simulink model "bh_test_LINCONT_on_NONLIN_plant"  (R2016a)
settings: Solver=ode23s  StartTime=0.0  StopTime=30  FixedStep=0.001  RelTol=1e-5
undefined symbols (not defined in the file or in its folder): P_one_prop, P_veh, sigbuilder_block
libraries: simulink x6, simulink_extras x5, bh_6dof_LIBRARY x2
settings Model: Creator=bhorton  LastModifiedBy=bhorton
settings DataIOCC: SaveOutput=off  SignalLogging=off  DSMLogging=off  VisualizeSimOutput=off  SaveTime=off
settings DebuggingCC: AllowSymbolicDim=off
settings ModelReferenceCC: PropagateSignalLabelsOutOfModel=off
settings GRTTargetCC: GeneratePreprocessorConditionals=Use local settings

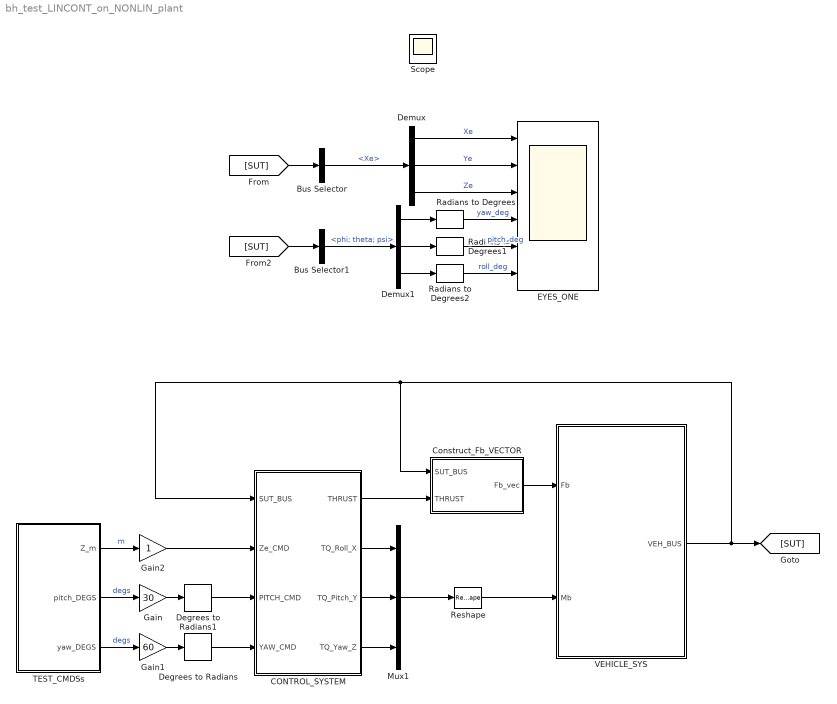
== system bh_test_LINCONT_on_NONLIN_plant ==
  Bus Selector : BusSelector  OutputSignals=Xe
  Bus Selector1 : BusSelector  OutputSignals=phi; theta; psi
  CONTROL_SYSTEM : Subsystem
  Construct_Fb_VECTOR : Subsystem
  Degrees to Radians : simulink_extras/Transformations/Degrees to Radians
  Degrees to Radians1 : simulink_extras/Transformations/Degrees to Radians
  Demux : Demux  Outputs=3
  Demux1 : Demux  Outputs=3
  EYES_ONE : Scope  NumInputPorts=6
  Gain : Gain  Gain=30
  Gain1 : Gain  Gain=60
  Gain2 : Gain
  Mux1 : Mux  Inputs=3
  Radians to Degrees : simulink_extras/Transformations/Radians to Degrees
  Radians to Degrees1 : simulink_extras/Transformations/Radians to Degrees
  Radians to Degrees2 : simulink_extras/Transformations/Radians to Degrees
  Reshape : Reshape  OutputDimensionality=Column vector (2-D)
  TEST_CMDSs : Subsystem  Tag=STV Subsys  LoadFcn=sigbuilder_block('load');  StartFcn=sigbuilder_block('start');  StopFcn=sigbuilder_block('stop');  ClipboardFcn=sigbuilder_block('clipboard');  mask(Sigbuilder block){}
      mask help: Simulink:masks:SigbuilderBlock_MD
      mask init:
      | if ~strcmp(get_param(bdroot(gcbh),'SimulationStatus'),'stopped') tuvar = sigbuilder_block('maskInit'); end
      settings: CopyFcn=sigbuilder_block('copy');  DeleteFcn=sigbuilder_block('delete');  ModelCloseFcn=sigbuilder_block('modelClose');  PreSaveFcn=sigbuilder_block('preSave');  PauseFcn=sigbuilder_block('pause');  ContinueFcn=sigbuilder_block('continue');  NameChangeFcn=sigbuilder_block('namechange');  OpenFcn=sigbuilder_block('open',[140.25 198.75 550.5 399.75 ]);  CloseFcn=sigbuilder_block('close');
      mask Display: plot(0, 0, 100, 100,[2, 2, 32, 32, 2], [68, 8, 8, 68, 68],[32, 2], [38, 38], [32, 19, 2],[53, 60, 44], [32, 17, 17, 2],[16, 16, 31, 31]);txt = getActiveGroup(gcbh);text(2, 100, txt,'verticalAlignment', 'top');
  VEHICLE_SYS : Subsystem
  Scope : Scope
  wires:
  Construct_Fb_VECTOR/1(Fb_vec) -> VEHICLE_SYS/1(Fb)
  Reshape/1 -> VEHICLE_SYS/2(Mb)
  Mux1/1 -> Reshape/1
  TEST_CMDSs/2(pitch_DEGS) -> Gain/1  "degs"
  TEST_CMDSs/1(Z_m) -> Gain2/1  "m"
  TEST_CMDSs/3(yaw_DEGS) -> Gain1/1  "degs"
  Gain/1 -> Degrees to Radians1/1
  Gain1/1 -> Degrees to Radians/1
  Degrees to Radians/1 -> CONTROL_SYSTEM/4(YAW_CMD)
  Degrees to Radians1/1 -> CONTROL_SYSTEM/3(PITCH_CMD)
  CONTROL_SYSTEM/1(THRUST) -> Construct_Fb_VECTOR/2(THRUST)
  CONTROL_SYSTEM/2(TQ_Roll_X) -> Mux1/1
  CONTROL_SYSTEM/3(TQ_Pitch_Y) -> Mux1/2
  CONTROL_SYSTEM/4(TQ_Yaw_Z) -> Mux1/3
  [SUT] -> Bus Selector/1
  Demux/2 -> EYES_ONE/2  "Ye"
  Demux/3 -> EYES_ONE/3  "Ze"
  Demux/1 -> EYES_ONE/1  "Xe"
  Bus Selector/1 -> Demux/1  "<Xe>"
  Bus Selector1/1 -> Demux1/1  "<phi; theta; psi>"
  [SUT] -> Bus Selector1/1
  Demux1/1 -> Radians to Degrees/1
  Radians to Degrees/1 -> EYES_ONE/4  "yaw_deg"
  Radians to Degrees1/1 -> EYES_ONE/5  "pitch_deg"
  Radians to Degrees2/1 -> EYES_ONE/6  "roll_deg"
  Demux1/3 -> Radians to Degrees2/1
  Demux1/2 -> Radians to Degrees1/1
  VEHICLE_SYS/1(VEH_BUS) -> [SUT], CONTROL_SYSTEM/1(SUT_BUS), Construct_Fb_VECTOR/1(SUT_BUS)
  Gain2/1 -> CONTROL_SYSTEM/2(Ze_CMD)

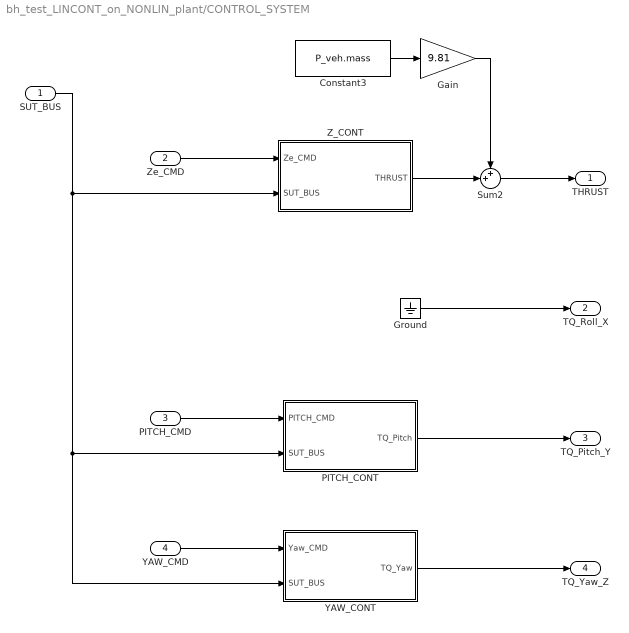
== system bh_test_LINCONT_on_NONLIN_plant/CONTROL_SYSTEM ==
  SUT_BUS : Inport
  Ze_CMD : Inport  Port=2
  PITCH_CMD : Inport  Port=3
  YAW_CMD : Inport  Port=4
  Constant3 : Constant  Value=P_veh.mass
  Gain : Gain  Gain=9.81
  Ground : Ground
  PITCH_CONT : Subsystem
  Sum2 : Sum  Inputs=++|
  YAW_CONT : Subsystem
  Z_CONT : Subsystem
  THRUST : Outport
  TQ_Roll_X : Outport  Port=2
  TQ_Pitch_Y : Outport  Port=3
  TQ_Yaw_Z : Outport  Port=4
  wires:
  SUT_BUS/1 -> PITCH_CONT/2(SUT_BUS), YAW_CONT/2(SUT_BUS), Z_CONT/2(SUT_BUS)
  Ze_CMD/1 -> Z_CONT/1(Ze_CMD)
  PITCH_CMD/1 -> PITCH_CONT/1(PITCH_CMD)
  YAW_CMD/1 -> YAW_CONT/1(Yaw_CMD)
  Z_CONT/1(THRUST) -> Sum2/2
  YAW_CONT/1(TQ_Yaw) -> TQ_Yaw_Z/1
  PITCH_CONT/1(TQ_Pitch) -> TQ_Pitch_Y/1
  Ground/1 -> TQ_Roll_X/1
  Sum2/1 -> THRUST/1
  Gain/1 -> Sum2/1
  Constant3/1 -> Gain/1

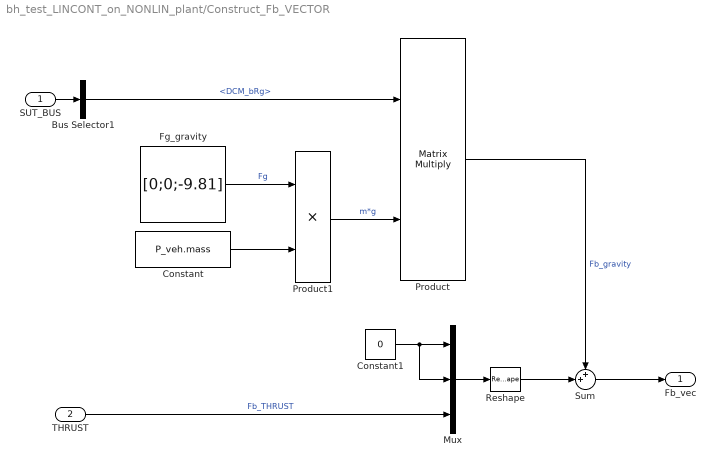
== system bh_test_LINCONT_on_NONLIN_plant/Construct_Fb_VECTOR ==
  SUT_BUS : Inport
  THRUST : Inport  Port=2
  Bus Selector1 : BusSelector  OutputSignals=DCM_bRg
  Constant : Constant  Value=P_veh.mass
  Constant1 : Constant  Value=0
  Fg_gravity : Constant  Value=[0;0;-9.81]  VectorParams1D=off
  Mux : Mux  Inputs=3
  Product : Product  Multiplication=Matrix(*)
  Product1 : Product
  Reshape : Reshape  OutputDimensionality=Column vector (2-D)
  Sum : Sum  Inputs=++|
  Fb_vec : Outport
  wires:
  Mux/1 -> Reshape/1
  Sum/1 -> Fb_vec/1
  SUT_BUS/1 -> Bus Selector1/1
  THRUST/1 -> Mux/3  "Fb_THRUST"
  Constant1/1 -> Mux/2, Mux/1
  Bus Selector1/1 -> Product/1  "<DCM_bRg>"
  Reshape/1 -> Sum/2
  Product/1 -> Sum/1  "Fb_gravity"
  Product1/1 -> Product/2  "m*g"
  Fg_gravity/1 -> Product1/1  "Fg"
  Constant/1 -> Product1/2

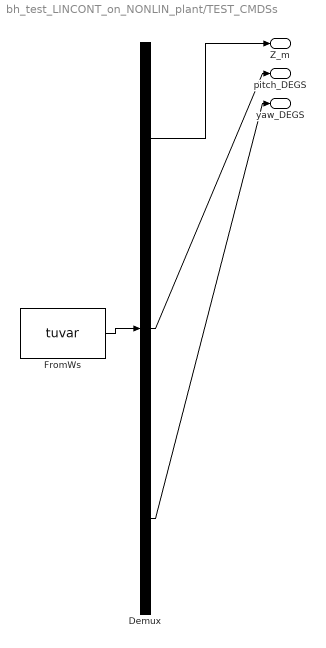
== system bh_test_LINCONT_on_NONLIN_plant/TEST_CMDSs ==
  Demux : Demux  Tag=STV Demux  Outputs=3
  FromWs : FromWorkspace  Tag=STV FromWs  VariableName=tuvar  SampleTime=0
      SigBuilderData=|
      | common.afterFinalStr = 'Extrapolate'
      | common.sampleTime = 0
      | dataSet.timeRange = [0 20]
      | dataSet.name = 'Group 1'
      | sbobj.Groups.Name = 'Group 1'
      | sbobj.Groups.Signals(1).Name = 'Z_m'
      | sbobj.Groups.Signals(1).XData = [0 1 1 6 20]
      | sbobj.Groups.Signals(1).YData = [0 0 1 1 1]
      | sbobj.Groups.Signals(2).Name = 'pitch_DEGS'
      | sbobj.Groups.Signals(2).XData = [0 8 8 10 10 20]
      | sbobj.Groups.Signals(2).YData = [0 0 1 1 0 0]
      | sbobj.Groups.Signals(3).Name = 'yaw_DEGS'
      | sbobj.Groups.Signals(3).XData = [0 13.95 13.95 18 18 20]
      | sbobj.Groups.Signals(3).YData = [0 0 1 1 0 0]
      | sbobj.Groups.TimeRange = [0 20]
  Z_m : Outport  Tag=STV Outport
  pitch_DEGS : Outport  Tag=STV Outport  Port=2
  yaw_DEGS : Outport  Tag=STV Outport  Port=3
  wires:
  Demux/1 -> Z_m/1
  FromWs/1 -> Demux/1
  Demux/2 -> pitch_DEGS/1
  Demux/3 -> yaw_DEGS/1

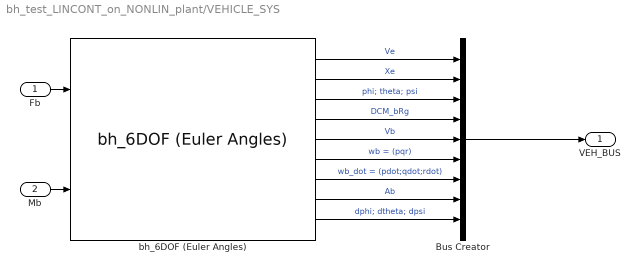
== system bh_test_LINCONT_on_NONLIN_plant/VEHICLE_SYS ==
  Fb : Inport
  Mb : Inport  Port=2
  Bus Creator : BusCreator  Inputs=9
  bh_6DOF (Euler Angles) : bh_6dof_LIBRARY/MODELS/bh_6DOF (Euler Angles)  inertia_0=P_veh.I  mass_0=P_veh.mass  xme_0=P_veh.Xe_init  Vm_0=P_veh.Vb_init  pm_0=P_veh.wb_init  eul_0=P_veh.eul_init
  VEH_BUS : Outport
  wires:
  Fb/1 -> bh_6DOF (Euler Angles)/1
  Mb/1 -> bh_6DOF (Euler Angles)/2
  bh_6DOF (Euler Angles)/3 -> Bus Creator/3  "phi; theta; psi"
  bh_6DOF (Euler Angles)/2 -> Bus Creator/2  "Xe"
  bh_6DOF (Euler Angles)/1 -> Bus Creator/1  "Ve"
  bh_6DOF (Euler Angles)/4 -> Bus Creator/4  "DCM_bRg"
  bh_6DOF (Euler Angles)/8 -> Bus Creator/8  "Ab"
  bh_6DOF (Euler Angles)/7 -> Bus Creator/7  "wb_dot = (pdot;qdot;rdot)"
  Bus Creator/1 -> VEH_BUS/1
  bh_6DOF (Euler Angles)/5 -> Bus Creator/5  "Vb"
  bh_6DOF (Euler Angles)/6 -> Bus Creator/6  "wb = (pqr)"
  bh_6DOF (Euler Angles)/9 -> Bus Creator/9  "dphi; dtheta; dpsi"

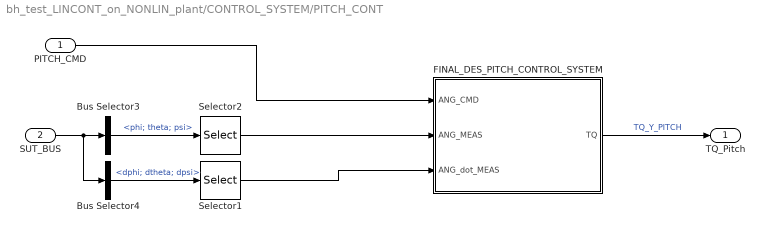
== system bh_test_LINCONT_on_NONLIN_plant/CONTROL_SYSTEM/PITCH_CONT ==
  PITCH_CMD : Inport
  SUT_BUS : Inport  Port=2
  Bus Selector3 : BusSelector  OutputSignals=phi; theta; psi
  Bus Selector4 : BusSelector  OutputSignals=dphi; dtheta; dpsi
  FINAL_DES_PITCH_CONTROL_SYSTEM : Subsystem
  Selector1 : Selector  InputPortWidth=3  IndexOptions=Index vector (dialog)  Indices=2  OutputSizes=1
  Selector2 : Selector  InputPortWidth=3  IndexOptions=Index vector (dialog)  Indices=2  OutputSizes=1
  TQ_Pitch : Outport
  wires:
  Selector2/1 -> FINAL_DES_PITCH_CONTROL_SYSTEM/2(ANG_MEAS)
  PITCH_CMD/1 -> FINAL_DES_PITCH_CONTROL_SYSTEM/1(ANG_CMD)
  Selector1/1 -> FINAL_DES_PITCH_CONTROL_SYSTEM/3(ANG_dot_MEAS)
  FINAL_DES_PITCH_CONTROL_SYSTEM/1(TQ) -> TQ_Pitch/1  "TQ_Y_PITCH"
  Bus Selector4/1 -> Selector1/1  "<dphi; dtheta; dpsi>"
  Bus Selector3/1 -> Selector2/1  "<phi; theta; psi>"
  SUT_BUS/1 -> Bus Selector4/1, Bus Selector3/1

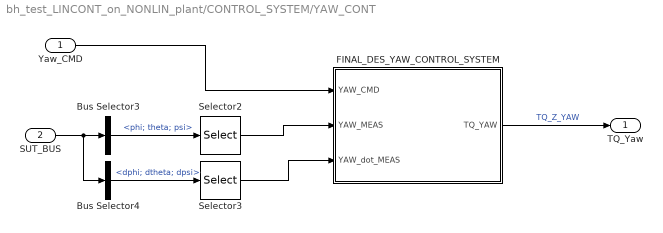
== system bh_test_LINCONT_on_NONLIN_plant/CONTROL_SYSTEM/YAW_CONT ==
  Yaw_CMD : Inport
  SUT_BUS : Inport  Port=2
  Bus Selector3 : BusSelector  OutputSignals=phi; theta; psi
  Bus Selector4 : BusSelector  OutputSignals=dphi; dtheta; dpsi
  FINAL_DES_YAW_CONTROL_SYSTEM : Subsystem
  Selector2 : Selector  InputPortWidth=3  IndexOptions=Index vector (dialog)  Indices=1  OutputSizes=1
  Selector3 : Selector  InputPortWidth=3  IndexOptions=Index vector (dialog)  Indices=1  OutputSizes=1
  TQ_Yaw : Outport
  wires:
  Selector2/1 -> FINAL_DES_YAW_CONTROL_SYSTEM/2(YAW_MEAS)
  Yaw_CMD/1 -> FINAL_DES_YAW_CONTROL_SYSTEM/1(YAW_CMD)
  Selector3/1 -> FINAL_DES_YAW_CONTROL_SYSTEM/3(YAW_dot_MEAS)
  FINAL_DES_YAW_CONTROL_SYSTEM/1(TQ_YAW) -> TQ_Yaw/1  "TQ_Z_YAW"
  Bus Selector4/1 -> Selector3/1  "<dphi; dtheta; dpsi>"
  Bus Selector3/1 -> Selector2/1  "<phi; theta; psi>"
  SUT_BUS/1 -> Bus Selector4/1, Bus Selector3/1

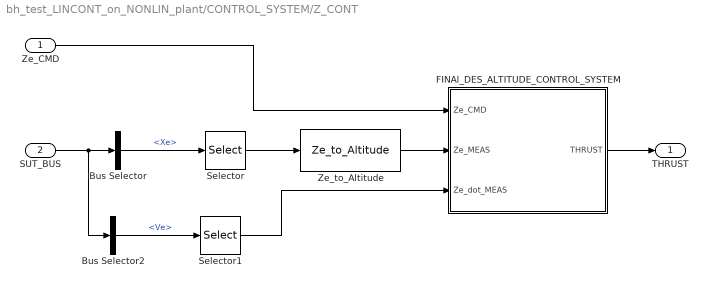
== system bh_test_LINCONT_on_NONLIN_plant/CONTROL_SYSTEM/Z_CONT ==
  Ze_CMD : Inport
  SUT_BUS : Inport  Port=2
  Bus Selector : BusSelector  OutputSignals=Xe
  Bus Selector2 : BusSelector  OutputSignals=Ve
  FINAl_DES_ALTITUDE_CONTROL_SYSTEM : Subsystem
  Selector : Selector  InputPortWidth=3  IndexOptions=Index vector (dialog)  Indices=3  OutputSizes=1
  Selector1 : Selector  InputPortWidth=3  IndexOptions=Index vector (dialog)  Indices=3  OutputSizes=1
  Ze_to_Altitude : bh_6dof_LIBRARY/MODELS/Ze_to_Altitude  SystemSampleTime=-1
  THRUST : Outport
  wires:
  Selector1/1 -> FINAl_DES_ALTITUDE_CONTROL_SYSTEM/3(Ze_dot_MEAS)
  Ze_to_Altitude/1 -> FINAl_DES_ALTITUDE_CONTROL_SYSTEM/2(Ze_MEAS)
  FINAl_DES_ALTITUDE_CONTROL_SYSTEM/1(THRUST) -> THRUST/1
  SUT_BUS/1 -> Bus Selector2/1, Bus Selector/1
  Ze_CMD/1 -> FINAl_DES_ALTITUDE_CONTROL_SYSTEM/1(Ze_CMD)
  Bus Selector2/1 -> Selector1/1  "<Ve>"
  Bus Selector/1 -> Selector/1  "<Xe>"
  Selector/1 -> Ze_to_Altitude/1

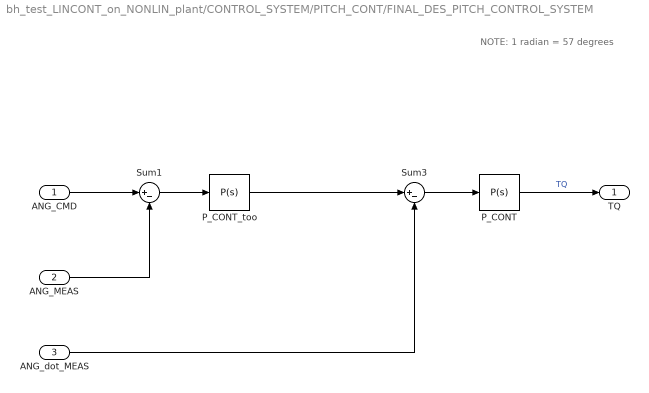
== system bh_test_LINCONT_on_NONLIN_plant/CONTROL_SYSTEM/PITCH_CONT/FINAL_DES_PITCH_CONTROL_SYSTEM ==
  note: NOTE: 1 radian = 57 degrees
  ANG_CMD : Inport
  ANG_MEAS : Inport  Port=2
  ANG_dot_MEAS : Inport  Port=3
  P_CONT : simulink/Continuous/PID Controller  Controller=P  TimeDomain=Continuous-time  SampleTime=-1  IntegratorMethod=Forward Euler  FilterMethod=Forward Euler  Form=Parallel  UseFilter=on  ControllerParametersSource=internal  P=0.0507941015552232  I=7.09690484808648  D=-0.334898279224841  N=17.076664592689  InitialConditionSource=internal  InitialConditionForIntegrator=0  InitialConditionForFilter=0  ExternalReset=none  LimitOutput=off  UpperSaturationLimit=inf  LowerSaturationLimit=-inf  LinearizeAsGain=on  AntiWindupMode=none  Kb=1  TrackingMode=off  Kt=1  PParamMin=[]  PParamMax=[]  IParamMin=[]  IParamMax=[]  DParamMin=[]  DParamMax=[]  NParamMin=[]  NParamMax=[]  KbParamMin=[]  KbParamMax=[]  KtParamMin=[]  KtParamMax=[]  POutMin=[]  POutMax=[]  IOutMin=[]  IOutMax=[]  DOutMin=[]  DOutMax=[]  NOutMin=[]  NOutMax=[]  KbOutMin=[]  KbOutMax=[]  KtOutMin=[]  KtOutMax=[]  IntegratorOutMin=[]  IntegratorOutMax=[]  FilterOutMin=[]  FilterOutMax=[]  SumOutMin=[]  SumOutMax=[]  SumI1OutMin=[]  SumI1OutMax=[]  SumI2OutMin=[]  SumI2OutMax=[]  SumI3OutMin=[]  SumI3OutMax=[]  SumDOutMin=[]  SumDOutMax=[]  SaturationOutMin=[]  SaturationOutMax=[]  IntegratorContinuousStateAttributes=''  IntegratorStateMustResolveToSignalObject=off  IntegratorRTWStateStorageClass=Auto  FilterContinuousStateAttributes=''  FilterStateMustResolveToSignalObject=off  FilterRTWStateStorageClass=Auto  DifferentiatorICPrevScaledInput=0  DifferentiatorOutMin=[]  DifferentiatorOutMax=[]
  P_CONT_too : simulink/Continuous/PID Controller  Controller=P  TimeDomain=Continuous-time  SampleTime=-1  IntegratorMethod=Forward Euler  FilterMethod=Forward Euler  Form=Parallel  UseFilter=on  ControllerParametersSource=internal  P=3.111442907298  I=0.151389824684851  D=0  N=100  InitialConditionSource=internal  InitialConditionForIntegrator=0  InitialConditionForFilter=0  ExternalReset=none  LimitOutput=off  UpperSaturationLimit=inf  LowerSaturationLimit=-inf  LinearizeAsGain=on  AntiWindupMode=none  Kb=1  TrackingMode=off  Kt=1  PParamMin=[]  PParamMax=[]  IParamMin=[]  IParamMax=[]  DParamMin=[]  DParamMax=[]  NParamMin=[]  NParamMax=[]  KbParamMin=[]  KbParamMax=[]  KtParamMin=[]  KtParamMax=[]  POutMin=[]  POutMax=[]  IOutMin=[]  IOutMax=[]  DOutMin=[]  DOutMax=[]  NOutMin=[]  NOutMax=[]  KbOutMin=[]  KbOutMax=[]  KtOutMin=[]  KtOutMax=[]  IntegratorOutMin=[]  IntegratorOutMax=[]  FilterOutMin=[]  FilterOutMax=[]  SumOutMin=[]  SumOutMax=[]  SumI1OutMin=[]  SumI1OutMax=[]  SumI2OutMin=[]  SumI2OutMax=[]  SumI3OutMin=[]  SumI3OutMax=[]  SumDOutMin=[]  SumDOutMax=[]  SaturationOutMin=[]  SaturationOutMax=[]  IntegratorContinuousStateAttributes=''  IntegratorStateMustResolveToSignalObject=off  IntegratorRTWStateStorageClass=Auto  FilterContinuousStateAttributes=''  FilterStateMustResolveToSignalObject=off  FilterRTWStateStorageClass=Auto  DifferentiatorICPrevScaledInput=0  DifferentiatorOutMin=[]  DifferentiatorOutMax=[]
  Sum1 : Sum  Inputs=|+-
  Sum3 : Sum  Inputs=|+-
  TQ : Outport
  wires:
  Sum3/1 -> P_CONT/1
  P_CONT/1 -> TQ/1  "TQ"
  ANG_MEAS/1 -> Sum1/2
  ANG_dot_MEAS/1 -> Sum3/2
  Sum1/1 -> P_CONT_too/1
  ANG_CMD/1 -> Sum1/1
  P_CONT_too/1 -> Sum3/1

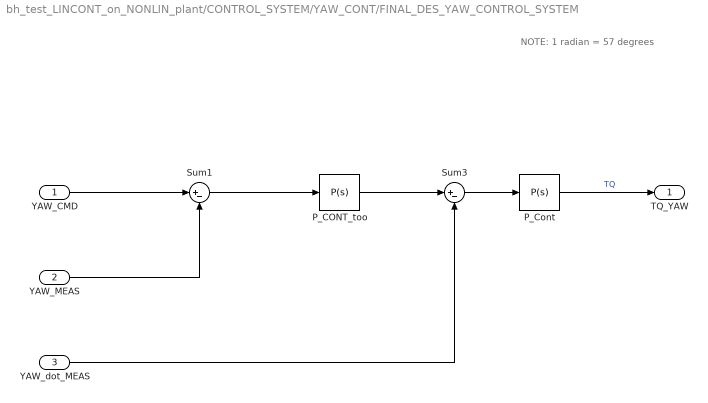
== system bh_test_LINCONT_on_NONLIN_plant/CONTROL_SYSTEM/YAW_CONT/FINAL_DES_YAW_CONTROL_SYSTEM ==
  note: NOTE: 1 radian = 57 degrees
  YAW_CMD : Inport
  YAW_MEAS : Inport  Port=2
  YAW_dot_MEAS : Inport  Port=3
  P_CONT_too : simulink/Continuous/PID Controller  Controller=P  TimeDomain=Continuous-time  SampleTime=-1  IntegratorMethod=Forward Euler  FilterMethod=Forward Euler  Form=Parallel  UseFilter=on  ControllerParametersSource=internal  P=1.61636567778084  I=0.151389824684851  D=0  N=100  InitialConditionSource=internal  InitialConditionForIntegrator=0  InitialConditionForFilter=0  ExternalReset=none  LimitOutput=off  UpperSaturationLimit=inf  LowerSaturationLimit=-inf  LinearizeAsGain=on  AntiWindupMode=none  Kb=1  TrackingMode=off  Kt=1  PParamMin=[]  PParamMax=[]  IParamMin=[]  IParamMax=[]  DParamMin=[]  DParamMax=[]  NParamMin=[]  NParamMax=[]  KbParamMin=[]  KbParamMax=[]  KtParamMin=[]  KtParamMax=[]  POutMin=[]  POutMax=[]  IOutMin=[]  IOutMax=[]  DOutMin=[]  DOutMax=[]  NOutMin=[]  NOutMax=[]  KbOutMin=[]  KbOutMax=[]  KtOutMin=[]  KtOutMax=[]  IntegratorOutMin=[]  IntegratorOutMax=[]  FilterOutMin=[]  FilterOutMax=[]  SumOutMin=[]  SumOutMax=[]  SumI1OutMin=[]  SumI1OutMax=[]  SumI2OutMin=[]  SumI2OutMax=[]  SumI3OutMin=[]  SumI3OutMax=[]  SumDOutMin=[]  SumDOutMax=[]  SaturationOutMin=[]  SaturationOutMax=[]  IntegratorContinuousStateAttributes=''  IntegratorStateMustResolveToSignalObject=off  IntegratorRTWStateStorageClass=Auto  FilterContinuousStateAttributes=''  FilterStateMustResolveToSignalObject=off  FilterRTWStateStorageClass=Auto  DifferentiatorICPrevScaledInput=0  DifferentiatorOutMin=[]  DifferentiatorOutMax=[]
  P_Cont : simulink/Continuous/PID Controller  Controller=P  TimeDomain=Continuous-time  SampleTime=-1  IntegratorMethod=Forward Euler  FilterMethod=Forward Euler  Form=Parallel  UseFilter=on  ControllerParametersSource=internal  P=0.09744859506471  I=7.09690484808648  D=-0.334898279224841  N=17.076664592689  InitialConditionSource=internal  InitialConditionForIntegrator=0  InitialConditionForFilter=0  ExternalReset=none  LimitOutput=off  UpperSaturationLimit=inf  LowerSaturationLimit=-inf  LinearizeAsGain=on  AntiWindupMode=none  Kb=1  TrackingMode=off  Kt=1  PParamMin=[]  PParamMax=[]  IParamMin=[]  IParamMax=[]  DParamMin=[]  DParamMax=[]  NParamMin=[]  NParamMax=[]  KbParamMin=[]  KbParamMax=[]  KtParamMin=[]  KtParamMax=[]  POutMin=[]  POutMax=[]  IOutMin=[]  IOutMax=[]  DOutMin=[]  DOutMax=[]  NOutMin=[]  NOutMax=[]  KbOutMin=[]  KbOutMax=[]  KtOutMin=[]  KtOutMax=[]  IntegratorOutMin=[]  IntegratorOutMax=[]  FilterOutMin=[]  FilterOutMax=[]  SumOutMin=[]  SumOutMax=[]  SumI1OutMin=[]  SumI1OutMax=[]  SumI2OutMin=[]  SumI2OutMax=[]  SumI3OutMin=[]  SumI3OutMax=[]  SumDOutMin=[]  SumDOutMax=[]  SaturationOutMin=[]  SaturationOutMax=[]  IntegratorContinuousStateAttributes=''  IntegratorStateMustResolveToSignalObject=off  IntegratorRTWStateStorageClass=Auto  FilterContinuousStateAttributes=''  FilterStateMustResolveToSignalObject=off  FilterRTWStateStorageClass=Auto  DifferentiatorICPrevScaledInput=0  DifferentiatorOutMin=[]  DifferentiatorOutMax=[]
  Sum1 : Sum  Inputs=|+-
  Sum3 : Sum  Inputs=|+-
  TQ_YAW : Outport
  wires:
  Sum3/1 -> P_Cont/1
  P_Cont/1 -> TQ_YAW/1  "TQ"
  YAW_CMD/1 -> Sum1/1
  YAW_MEAS/1 -> Sum1/2
  YAW_dot_MEAS/1 -> Sum3/2
  Sum1/1 -> P_CONT_too/1
  P_CONT_too/1 -> Sum3/1

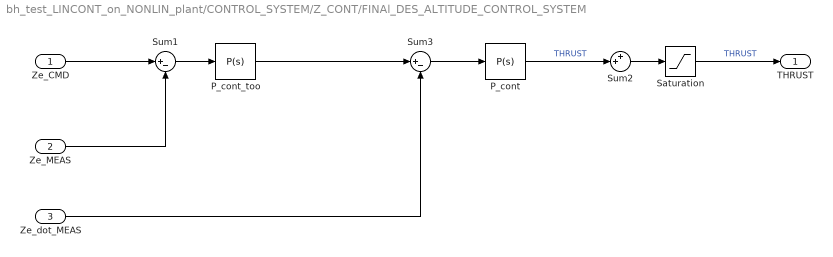
== system bh_test_LINCONT_on_NONLIN_plant/CONTROL_SYSTEM/Z_CONT/FINAl_DES_ALTITUDE_CONTROL_SYSTEM ==
  Ze_CMD : Inport
  Ze_MEAS : Inport  Port=2
  Ze_dot_MEAS : Inport  Port=3
  P_cont : simulink/Continuous/PID Controller  Controller=P  TimeDomain=Continuous-time  SampleTime=-1  IntegratorMethod=Forward Euler  FilterMethod=Forward Euler  Form=Parallel  UseFilter=on  ControllerParametersSource=internal  P=6.7862699178667  I=7.09690484808648  D=-0.334898279224841  N=17.076664592689  InitialConditionSource=internal  InitialConditionForIntegrator=0  InitialConditionForFilter=0  ExternalReset=none  LimitOutput=off  UpperSaturationLimit=inf  LowerSaturationLimit=-inf  LinearizeAsGain=on  AntiWindupMode=none  Kb=1  TrackingMode=off  Kt=1  PParamMin=[]  PParamMax=[]  IParamMin=[]  IParamMax=[]  DParamMin=[]  DParamMax=[]  NParamMin=[]  NParamMax=[]  KbParamMin=[]  KbParamMax=[]  KtParamMin=[]  KtParamMax=[]  POutMin=[]  POutMax=[]  IOutMin=[]  IOutMax=[]  DOutMin=[]  DOutMax=[]  NOutMin=[]  NOutMax=[]  KbOutMin=[]  KbOutMax=[]  KtOutMin=[]  KtOutMax=[]  IntegratorOutMin=[]  IntegratorOutMax=[]  FilterOutMin=[]  FilterOutMax=[]  SumOutMin=[]  SumOutMax=[]  SumI1OutMin=[]  SumI1OutMax=[]  SumI2OutMin=[]  SumI2OutMax=[]  SumI3OutMin=[]  SumI3OutMax=[]  SumDOutMin=[]  SumDOutMax=[]  SaturationOutMin=[]  SaturationOutMax=[]  IntegratorContinuousStateAttributes=''  IntegratorStateMustResolveToSignalObject=off  IntegratorRTWStateStorageClass=Auto  FilterContinuousStateAttributes=''  FilterStateMustResolveToSignalObject=off  FilterRTWStateStorageClass=Auto  DifferentiatorICPrevScaledInput=0  DifferentiatorOutMin=[]  DifferentiatorOutMax=[]
  P_cont_too : simulink/Continuous/PID Controller  Controller=P  TimeDomain=Continuous-time  SampleTime=-1  IntegratorMethod=Forward Euler  FilterMethod=Forward Euler  Form=Parallel  UseFilter=on  ControllerParametersSource=internal  P=0.931782439164433  I=0.151389824684851  D=0.117353405685993  N=2.94633103429336  InitialConditionSource=internal  InitialConditionForIntegrator=0  InitialConditionForFilter=0  ExternalReset=none  LimitOutput=off  UpperSaturationLimit=inf  LowerSaturationLimit=-inf  LinearizeAsGain=on  AntiWindupMode=none  Kb=1  TrackingMode=off  Kt=1  PParamMin=[]  PParamMax=[]  IParamMin=[]  IParamMax=[]  DParamMin=[]  DParamMax=[]  NParamMin=[]  NParamMax=[]  KbParamMin=[]  KbParamMax=[]  KtParamMin=[]  KtParamMax=[]  POutMin=[]  POutMax=[]  IOutMin=[]  IOutMax=[]  DOutMin=[]  DOutMax=[]  NOutMin=[]  NOutMax=[]  KbOutMin=[]  KbOutMax=[]  KtOutMin=[]  KtOutMax=[]  IntegratorOutMin=[]  IntegratorOutMax=[]  FilterOutMin=[]  FilterOutMax=[]  SumOutMin=[]  SumOutMax=[]  SumI1OutMin=[]  SumI1OutMax=[]  SumI2OutMin=[]  SumI2OutMax=[]  SumI3OutMin=[]  SumI3OutMax=[]  SumDOutMin=[]  SumDOutMax=[]  SaturationOutMin=[]  SaturationOutMax=[]  IntegratorContinuousStateAttributes=''  IntegratorStateMustResolveToSignalObject=off  IntegratorRTWStateStorageClass=Auto  FilterContinuousStateAttributes=''  FilterStateMustResolveToSignalObject=off  FilterRTWStateStorageClass=Auto  DifferentiatorICPrevScaledInput=0  DifferentiatorOutMin=[]  DifferentiatorOutMax=[]
  Saturation : Saturate  UpperLimit=4*P_one_prop.thrust_max  LowerLimit=-Inf
  Sum1 : Sum  Inputs=|+-
  Sum2 : Sum  Inputs=++|
  Sum3 : Sum  Inputs=|+-
  THRUST : Outport
  wires:
  ? -> Sum2/1
  Sum1/1 -> P_cont_too/1
  Sum3/1 -> P_cont/1
  Ze_CMD/1 -> Sum1/1
  Sum2/1 -> Saturation/1
  P_cont/1 -> Sum2/2  "THRUST"
  Saturation/1 -> THRUST/1  "THRUST"
  P_cont_too/1 -> Sum3/1
  Ze_MEAS/1 -> Sum1/2
  Ze_dot_MEAS/1 -> Sum3/2
